simulink model "PMSM_temperature_estimation_EKF"  (R2023b)
settings: Solver=VariableStepAuto  StartTime=0.0  StopTime=10  FixedStep=dt  RelTol=1e-3  AbsTol=1e-3
values from neighbouring files (symbols this model uses):
  CF_fc = 1/(20*Ts)    (= 5)    [controller_parameters.m]
  CF_k = 1    [controller_parameters.m]
  dt = 50e-6    (= 5e-05)    [config.m]
  dt_speed_control = 0.001    [config.m]
  max_power = 50e3    (= 50000)    [config.m]
  max_torque = 220    [config.m]
  N = 6    [config.m]
  ratio_rotor = 0.75    [config.m]
  Rd_percent_rotor = ratio_rotor*100    (= 75)    [config.m]
  Rm_percent_rotor = ratio_rotor*100    (= 75)    [config.m]
  rotor_initial_temperatures = 298.15    [config.m]
  stator_initial_temperatures = [298.15;298.15;298.15]    [config.m]
  stator_thermal_mass = 100    [config.m]
  Ts = 0.01    [controller_parameters.m]
undefined symbols (not defined in the file or in its folder): cex, ch, cJ, DiscIntNeverNeededParam
libraries: fl_lib x152, nesl_utility x45, fl_ps_legacy_lib x3, sharedTrackingLibrary x1, ee_lib x1, SignalEditorBlockLib x1, simulink x1
(part 3 of 3)

== system PMSM_temperature_estimation_EKF/Thermal Model/Sensing Temperature Rot ==
  PS-Simulink Converter : nesl_utility/PS-Simulink Converter  PhysicalDomain=network_engine_domain  SubClassName=ps_output  LeftPortType=input  RightPortType=output  PseudoPeriodic=off  Frequencies=[]  VectorFormat=1-D array  Unit=degC  AffineConversion=on
  Temperature Sensor : fl_lib/Thermal/Thermal Sensors/Temperature Sensor  temperature_measure=foundation.enum.MeasurementReference.difference
  ThRef : fl_lib/Thermal/Thermal Elements/Thermal Reference
  H : PMIOPort  Side=Left
  tag scope: TR=global
  wires:
  PS-Simulink Converter/1 -> [TR]
  connections:
  Temperature Sensor/RConn2 -- PS-Simulink Converter/LConn1
  ThRef/LConn1 -- Temperature Sensor/RConn1
  H/RConn1 -- Temperature Sensor/LConn1

== system PMSM_temperature_estimation_EKF/Thermal Model/Sensing Temperature WiA ==
  PS-Simulink Converter : nesl_utility/PS-Simulink Converter  PhysicalDomain=network_engine_domain  SubClassName=ps_output  LeftPortType=input  RightPortType=output  PseudoPeriodic=off  Frequencies=[]  VectorFormat=1-D array  Unit=degC  AffineConversion=on
  Temperature Sensor : fl_lib/Thermal/Thermal Sensors/Temperature Sensor  temperature_measure=foundation.enum.MeasurementReference.difference
  ThRef : fl_lib/Thermal/Thermal Elements/Thermal Reference
  H : PMIOPort  Side=Left
  tag scope: TA=global
  wires:
  PS-Simulink Converter/1 -> [TA]
  connections:
  H/RConn1 -- Temperature Sensor/LConn1
  ThRef/LConn1 -- Temperature Sensor/RConn1
  Temperature Sensor/RConn2 -- PS-Simulink Converter/LConn1

== system PMSM_temperature_estimation_EKF/Thermal Model/Sensing Temperature WiB ==
  PS-Simulink Converter : nesl_utility/PS-Simulink Converter  PhysicalDomain=network_engine_domain  SubClassName=ps_output  LeftPortType=input  RightPortType=output  PseudoPeriodic=off  Frequencies=[]  VectorFormat=1-D array  Unit=degC  AffineConversion=on
  Temperature Sensor : fl_lib/Thermal/Thermal Sensors/Temperature Sensor  temperature_measure=foundation.enum.MeasurementReference.difference
  ThRef : fl_lib/Thermal/Thermal Elements/Thermal Reference
  H : PMIOPort  Side=Left
  tag scope: TB=global
  wires:
  PS-Simulink Converter/1 -> [TB]
  connections:
  Temperature Sensor/RConn2 -- PS-Simulink Converter/LConn1
  ThRef/LConn1 -- Temperature Sensor/RConn1
  H/RConn1 -- Temperature Sensor/LConn1

== system PMSM_temperature_estimation_EKF/Thermal Model/Sensing Temperature WiC ==
  PS-Simulink Converter : nesl_utility/PS-Simulink Converter  PhysicalDomain=network_engine_domain  SubClassName=ps_output  LeftPortType=input  RightPortType=output  PseudoPeriodic=off  Frequencies=[]  VectorFormat=1-D array  Unit=degC  AffineConversion=on
  Temperature Sensor : fl_lib/Thermal/Thermal Sensors/Temperature Sensor  temperature_measure=foundation.enum.MeasurementReference.difference
  ThRef : fl_lib/Thermal/Thermal Elements/Thermal Reference
  H : PMIOPort  Side=Left
  tag scope: TC=global
  wires:
  PS-Simulink Converter/1 -> [TC]
  connections:
  H/RConn1 -- Temperature Sensor/LConn1
  ThRef/LConn1 -- Temperature Sensor/RConn1
  Temperature Sensor/RConn2 -- PS-Simulink Converter/LConn1

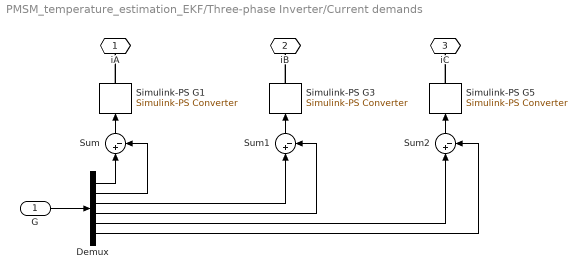
== system PMSM_temperature_estimation_EKF/Three-phase Inverter/Current demands ==
  G : Inport
  Demux : Demux  Outputs=[1,1,1,1,1,1]
  Simulink-PS G1 : nesl_utility/Simulink-PS Converter  PhysicalDomain=network_engine_domain  SubClassName=ps_input  LeftPortType=input  RightPortType=output  PseudoPeriodic=off  Frequencies=[]  NoiseDistribution=none  NoiseParameters=[]  Unit=1  AffineConversion=off  FilteringAndDerivatives=zero  SimscapeFilterOrder=1  InputFilterTimeConstant=1e-6  UdotUserProvided=1
  Simulink-PS G3 : nesl_utility/Simulink-PS Converter  PhysicalDomain=network_engine_domain  SubClassName=ps_input  LeftPortType=input  RightPortType=output  PseudoPeriodic=off  Frequencies=[]  NoiseDistribution=none  NoiseParameters=[]  Unit=1  AffineConversion=off  FilteringAndDerivatives=zero  SimscapeFilterOrder=1  InputFilterTimeConstant=1e-6  UdotUserProvided=0
  Simulink-PS G5 : nesl_utility/Simulink-PS Converter  PhysicalDomain=network_engine_domain  SubClassName=ps_input  LeftPortType=input  RightPortType=output  PseudoPeriodic=off  Frequencies=[]  NoiseDistribution=none  NoiseParameters=[]  Unit=1  AffineConversion=off  FilteringAndDerivatives=zero  SimscapeFilterOrder=1  InputFilterTimeConstant=1e-6  UdotUserProvided=0
  Sum : Sum  Inputs=|+-  InputSameDT=on  SaturateOnIntegerOverflow=on  OutDataTypeStr=Inherit: Same as first input
  Sum1 : Sum  Inputs=|+-  InputSameDT=on  SaturateOnIntegerOverflow=on  OutDataTypeStr=Inherit: Same as first input
  Sum2 : Sum  Inputs=|+-  InputSameDT=on  SaturateOnIntegerOverflow=on  OutDataTypeStr=Inherit: Same as first input
  iA : PMIOPort  Side=Right
  iB : PMIOPort  Port=2  Side=Right
  iC : PMIOPort  Port=3  Side=Right
  wires:
  G/1 -> Demux/1
  Demux/4 -> Sum1/2
  Demux/3 -> Sum1/1
  Demux/6 -> Sum2/2
  Sum1/1 -> Simulink-PS G3/1
  Demux/2 -> Sum/2
  Demux/5 -> Sum2/1
  Sum2/1 -> Simulink-PS G5/1
  Sum/1 -> Simulink-PS G1/1
  Demux/1 -> Sum/1
  connections:
  Simulink-PS G1/RConn1 -- iA/RConn1
  Simulink-PS G5/RConn1 -- iC/RConn1
  Simulink-PS G3/RConn1 -- iB/RConn1

== system PMSM_temperature_estimation_EKF/Three-phase Inverter/iA ==
  ERef : fl_lib/Electrical/Electrical Elements/Electrical Reference
  PS Product : fl_ps_legacy_lib/Legacy Physical Signals/Functions/PS Product
  Resistor : fl_lib/Electrical/Electrical Elements/Resistor  R=1000 Ohm  i_specify=off  i_priority=High  i=0 A  i_nominal_specify=off  i_nominal_unit=A  i_nominal_value=1  v_specify=off  v_priority=High  v=0 V  v_nominal_specify=off  v_nominal_unit=V  v_nominal_value=1
  Voltage Sensor : fl_lib/Electrical/Electrical Sensors/Voltage Sensor
  iA : fl_lib/Electrical/Electrical Sources/Controlled Current Source
  + : PMIOPort  Side=Right
  P : PMIOPort  Port=2  Side=Right
  ref : PMIOPort  Port=3  Side=Left
  connections:
  iA/LConn1 -- +/RConn1 -- Resistor/RConn1 -- Voltage Sensor/LConn1
  Voltage Sensor/RConn1 -- PS Product/LConn1
  PS Product/RConn1 -- P/RConn1
  ERef/LConn1 -- Resistor/LConn1 -- Voltage Sensor/RConn2 -- iA/RConn2
  iA/RConn1 -- PS Product/LConn2 -- ref/RConn1

== system PMSM_temperature_estimation_EKF/Three-phase Inverter/iB ==
  ERef : fl_lib/Electrical/Electrical Elements/Electrical Reference
  PS Product : fl_ps_legacy_lib/Legacy Physical Signals/Functions/PS Product
  Resistor : fl_lib/Electrical/Electrical Elements/Resistor  R=1000 Ohm  i_specify=off  i_priority=High  i=0 A  i_nominal_specify=off  i_nominal_unit=A  i_nominal_value=1  v_specify=off  v_priority=High  v=0 V  v_nominal_specify=off  v_nominal_unit=V  v_nominal_value=1
  Voltage Sensor : fl_lib/Electrical/Electrical Sensors/Voltage Sensor
  iA : fl_lib/Electrical/Electrical Sources/Controlled Current Source
  + : PMIOPort  Side=Right
  P : PMIOPort  Port=2  Side=Right
  ref : PMIOPort  Port=3  Side=Left
  connections:
  ref/RConn1 -- PS Product/LConn2 -- iA/RConn1
  Resistor/LConn1 -- Voltage Sensor/RConn2 -- iA/RConn2 -- ERef/LConn1
  PS Product/RConn1 -- P/RConn1
  Voltage Sensor/RConn1 -- PS Product/LConn1
  +/RConn1 -- Voltage Sensor/LConn1 -- Resistor/RConn1 -- iA/LConn1

== system PMSM_temperature_estimation_EKF/Three-phase Inverter/iC ==
  ERef : fl_lib/Electrical/Electrical Elements/Electrical Reference
  PS Product : fl_ps_legacy_lib/Legacy Physical Signals/Functions/PS Product
  Resistor : fl_lib/Electrical/Electrical Elements/Resistor  R=1000 Ohm  i_specify=off  i_priority=High  i=0 A  i_nominal_specify=off  i_nominal_unit=A  i_nominal_value=1  v_specify=off  v_priority=High  v=0 V  v_nominal_specify=off  v_nominal_unit=V  v_nominal_value=1
  Voltage Sensor : fl_lib/Electrical/Electrical Sensors/Voltage Sensor
  iA : fl_lib/Electrical/Electrical Sources/Controlled Current Source
  + : PMIOPort  Side=Right
  P : PMIOPort  Port=2  Side=Right
  ref : PMIOPort  Port=3  Side=Left
  connections:
  iA/LConn1 -- Resistor/RConn1 -- Voltage Sensor/LConn1 -- +/RConn1
  Voltage Sensor/RConn1 -- PS Product/LConn1
  PS Product/RConn1 -- P/RConn1
  ERef/LConn1 -- iA/RConn2 -- Voltage Sensor/RConn2 -- Resistor/LConn1
  iA/RConn1 -- PS Product/LConn2 -- ref/RConn1

== system PMSM_temperature_estimation_EKF/PMSM Controller/Vector controller/Current control and gate assignment (averaged) ==
  iRefABC : Inport
  iABC : Inport  Port=2
  Controlled current source assignments : Subsystem
  Terminator : Terminator
  G : Outport  VectorParamsAs1DForOutWhenUnconnected=off
  wires:
  Controlled current source assignments/1(G) -> G/1
  iABC/1 -> Terminator/1
  iRefABC/1 -> Controlled current source assignments/1(iRefABC)

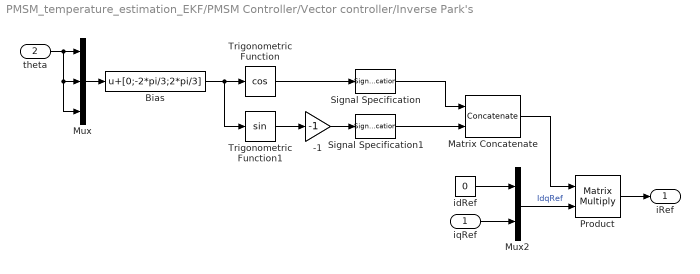
== system PMSM_temperature_estimation_EKF/PMSM Controller/Vector controller/Inverse Park's ==
  iqRef : Inport
  theta : Inport  Port=2
  -1 : Gain  Gain=-1  SaturateOnIntegerOverflow=on  OutDataTypeStr=Inherit: Same as input  ParamDataTypeStr=Inherit: Same as input
  Bias : Bias  Bias=[0;-2*pi/3;2*pi/3]  SaturateOnIntegerOverflow=off
  Matrix Concatenate : Concatenate  Mode=Multidimensional array  ConcatenateDimension=2
  Mux : Mux  Inputs=3
  Mux2 : Mux  Inputs=2
  Product : Product  Multiplication=Matrix(*)  RndMeth=Zero
  Signal Specification : SignalSpecification  Dimensions=[3 1]
  Signal Specification1 : SignalSpecification  Dimensions=[3 1]
  Trigonometric Function : Trigonometry  Operator=cos
  Trigonometric Function1 : Trigonometry
  idRef : Constant  Value=0  SampleTime=dt
  iRef : Outport  InitialOutput=0  VectorParamsAs1DForOutWhenUnconnected=off
  wires:
  -1/1 -> Signal Specification1/1
  Trigonometric Function/1 -> Signal Specification/1
  Product/1 -> iRef/1
  theta/1 -> Mux/1, Mux/2, Mux/3
  Bias/1 -> Trigonometric Function1/1, Trigonometric Function/1
  Trigonometric Function1/1 -> -1/1
  Signal Specification1/1 -> Matrix Concatenate/2
  Signal Specification/1 -> Matrix Concatenate/1
  idRef/1 -> Mux2/1
  iqRef/1 -> Mux2/2
  Mux2/1 -> Product/2  "IdqRef"
  Matrix Concatenate/1 -> Product/1
  Mux/1 -> Bias/1

== system PMSM_temperature_estimation_EKF/Speed Controller/Speed controller/Speed controller ==
  wRef : Inport
  wMeas : Inport  Port=2
  Add : Sum  Inputs=|+-
  Add1 : Sum
  Discrete-Time Integrator : DiscreteIntegrator  gainval=Ki  SampleTime=ts  LimitOutput=on  UpperSaturationLimit=trqMax  LowerSaturationLimit=-trqMax  ICPrevOutput=DiscIntNeverNeededParam  ICPrevScaledInput=DiscIntNeverNeededParam
  Kp : Gain  Gain=Kp
  trqRef : Outport  VectorParamsAs1DForOutWhenUnconnected=off
  wires:
  Add/1 -> Discrete-Time Integrator/1, Kp/1
  wMeas/1 -> Add/2
  Discrete-Time Integrator/1 -> Add1/2
  Kp/1 -> Add1/1
  wRef/1 -> Add/1
  Add1/1 -> trqRef/1

== system PMSM_temperature_estimation_EKF/PMSM Controller/Vector controller/Current control and gate assignment (averaged)/Controlled current source assignments ==
  iRefABC : Inport
  Constant : Constant  Value=[0;0;0]
  Constant1 : Constant  Value=[0;0;0]
  Demux : Demux  Outputs=3
  Demux1 : Demux  Outputs=3
  Gain : Gain  Gain=-1
  Mux : Mux  Inputs=6
  Switch : Switch  Criteria=u2 > Threshold  SaturateOnIntegerOverflow=off  InputSameDT=off
  Switch1 : Switch  Criteria=u2 > Threshold  SaturateOnIntegerOverflow=off  InputSameDT=off
  G : Outport  VectorParamsAs1DForOutWhenUnconnected=off
  wires:
  Demux1/1 -> Mux/2  "A(low)"
  Demux1/2 -> Mux/4  "B(low)"
  Demux/2 -> Mux/3  "B(high)"
  Demux/1 -> Mux/1  "A(high)"
  iRefABC/1 -> Switch/1, Switch/2, Gain/1
  Mux/1 -> G/1
  Demux1/3 -> Mux/6  "C(low)"
  Demux/3 -> Mux/5  "C(high)"
  Switch/1 -> Demux/1
  Switch1/1 -> Demux1/1
  Gain/1 -> Switch1/1, Switch1/2
  Constant/1 -> Switch/3
  Constant1/1 -> Switch1/3

== matlab function PMSM_temperature_estimation_EKF/park_transform ==
  data: Iabc input size=3; Idq output size=2; th input size=1
function Idq = park_transform(Iabc,th)
    Idq = sqrt(2/3)*[
        cos(th),cos(th-2*pi/3),cos(th+2*pi/3);
        -sin(th),-sin(th-2*pi/3),-sin(th+2*pi/3);
        ]*Iabc;
end

== matlab function PMSM_temperature_estimation_EKF/complementary_filter ==
  data: Iabc input size=3; Iabc output size=3; Ia input size=1; f input size=1; CF_k parameter; CF_fc parameter
function Iabc = complementary_filter(Iabc,Ia,f,CF_k, CF_fc)
    k = CF_k;
    fc = CF_fc;

    Iabc = 1/(1+exp(4*k*(f-fc)))*Iabc...
        +1/(1+exp(-4*k*(f-fc)))*[1;1;1]*Ia/sqrt(3);
end

== matlab function PMSM_temperature_estimation_EKF/State Space Model/MATLAB Function ==
  data: x input; u input; dxdt output
function dxdt = state_equation(x,u)
    dxdt = state_equation(x,u);
end

== matlab function PMSM_temperature_estimation_EKF/iron_loss ==
  data: f input size=1; Pall output size=1; Ia input size=1; ch parameter; cJ parameter; cex parameter
function Pall = iron_loss(f,Ia,ch,cJ,cex)
    Pall = iron_loss(f,Ia,ch,cJ,cex);
end

== matlab function PMSM_temperature_estimation_EKF/inverse_park_transform ==
  data: Idq input size=2; Iabc output size=3; th input size=1
function Iabc = inverse_park_transform(Idq,th)
    Iabc = sqrt(2/3)*[
        cos(th),cos(th-2*pi/3),cos(th+2*pi/3);
        -sin(th),-sin(th-2*pi/3),-sin(th+2*pi/3);
        ]'*Idq;
end
